simulink model "car_turning_state"  (R2020a)
settings: Solver=VariableStepAuto  StartTime=0.0  StopTime=10.0  RelTol=1e-3
settings Model: Creator=naina  LastModifiedBy=naina

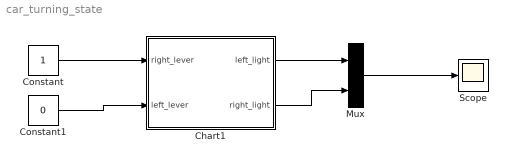
== system car_turning_state ==
  Chart1 : Stateflow chart  TreatAsAtomicUnit=on
  Constant : Constant
  Constant1 : Constant  Value=0
  Mux : Mux  Inputs=2
  Scope : Scope
  wires:
  Chart1/1(left_light) -> Mux/1
  Chart1/2(right_light) -> Mux/2
  Mux/1 -> Scope/1
  Constant/1 -> Chart1/1(right_lever)
  Constant1/1 -> Chart1/2(left_lever)

== stateflow chart car_turning_state/Chart1 ==
  state OFF
    entry:
    left_light = 0;
    right_light = 0;
  state LEFT
    state ON
      entry:
      left_light=1;
    state OFF
      entry:
      left_light=0;
    (default) -> LEFT.ON
    LEFT.OFF -> LEFT.ON : after(0.5,sec)
    LEFT.ON -> LEFT.OFF : after(0.5,sec)
  state RIGHT
    state ON
      entry:
      right_light=1;
    state OFF
      entry:
      right_light=0;
    (default) -> RIGHT.ON
    RIGHT.OFF -> RIGHT.ON : after(0.5,sec)
    RIGHT.ON -> RIGHT.OFF : after(0.5,sec)
  (default) -> OFF
  OFF -> RIGHT [order 1] : [right_lever == 1&left_lever == 0]
  OFF -> LEFT [order 2] : [right_lever == 0&left_lever == 1]
  LEFT -> OFF : [right_lever == 0&left_lever == 0]
  RIGHT -> OFF : [right_lever == 0&left_lever == 0]
  data: right_lever input; left_lever input; left_light output; right_light output
